simulink model "net2"  (R2014b)
settings: Solver=ode23tb  SolverMode=SingleTasking  StartTime=0.0  StopTime=0.06  RelTol=1e-4
libraries: powerlib x14
Description:
  | Copyright 2008-2014 The MathWorks, Inc.
settings Model: ExtModeTrigMode=oneshot  ExtModeArmWhenConnect=off  ExtModeAutoUpdateStatusClock=off  Creator=MathWorks  LastModifiedBy=jmmauricio
settings SolverCC: ZeroCrossAlgorithm=Adaptive
settings DataIOCC: LimitDataPoints=off  SignalLoggingSaveFormat=ModelDataLogs  SignalLoggingName=sigsOut
settings OptimizationCC: BooleanDataType=off  ExpressionDepthLimit=2147483647  InitFltsAndDblsToZero=on  EfficientMapNaN2IntZero=off
settings DebuggingCC: SaveWithParameterizedLinksMsg=none  UnderspecifiedInitializationDetection=Classic  MergeDetectMultiDrivingBlocksExec=none  SignalResolutionControl=TryResolveAllWithWarning  SolverPrmCheckMsg=none  MultiTaskDSMMsg=warning  MultiTaskCondExecSysMsg=none  SigSpecEnsureSampleTimeMsg=none  FcnCallInpInsideContextMsg=UseLocalSettings  StateNameClashWarn=warning
settings HardwareCC: TargetUnknown=on
settings RTWCC: IncludeERTFirstTime=on
settings GRTTargetCC: TargetFcnLib=ansi_tfl_tmw.mat  CombineOutputUpdateFcns=off  GRTInterface=on

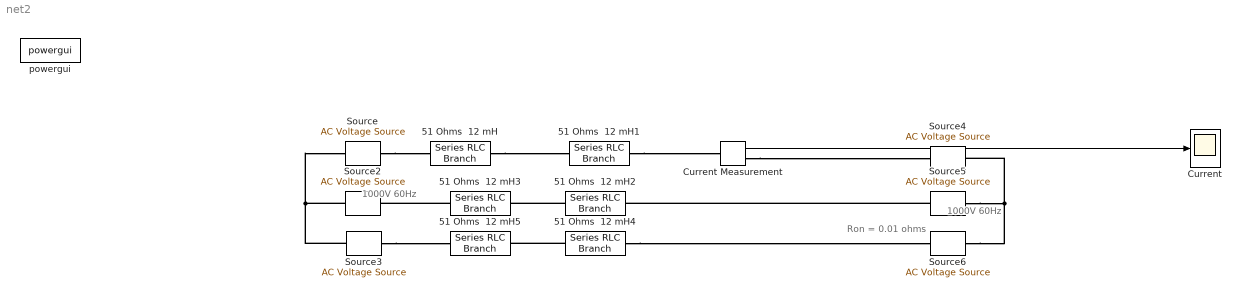
== system net2 ==
  note: Ron = 0.01 ohms
  note: 1000V
      |  60Hz
  note: 1000V
      |  60Hz
  51 Ohms  12 mH{,1..2,5} (4 alike) : powerlib/Elements/Series RLC Branch  LConnTagsString=__new0  RConnTagsString=__new0  BranchType=RL  Resistance=51  Inductance=12e-03  SetiL0=off  InitialCurrent=0  Capacitance=[]  Setx0=off  InitialVoltage=0  Measurements=None
  51 Ohms  12 mH3 : powerlib/Elements/Series RLC Branch  LConnTagsString=__new0  RConnTagsString=__new0  BranchType=RL  Resistance=2  Inductance=12e-03  SetiL0=off  InitialCurrent=0  Capacitance=[]  Setx0=off  InitialVoltage=0  Measurements=None
  51 Ohms  12 mH4 : powerlib/Elements/Series RLC Branch  LConnTagsString=__new0  RConnTagsString=__new0  BranchType=RL  Resistance=51  Inductance=50e-03  SetiL0=off  InitialCurrent=0  Capacitance=[]  Setx0=off  InitialVoltage=0  Measurements=None
  Current : Scope
      settings: TickLabels=on  TimeRange=0.06  YMin=-20  YMax=20
  Current Measurement : powerlib/Measurements/Current Measurement  Tag=PoWeRsYsTeMmEaSuReMeNt  PhasorSimulation=off  OutputType=Magnitude  PSBequivalent=0
  Source{,2..6} (6 alike) : powerlib/Electrical Sources/AC Voltage Source  Description=source block  Amplitude=1000  Phase=0  Frequency=60  SampleTime=0  Measurements=None
      settings: AttributesFormatString=\n
  powergui : powerlib/powergui  SimulationMode=Continuous  SolverType=Tustin  SampleTime=0  frequency=60  SPID=off  DisableSnubberDevices=off  DisableRonSwitches=off  DisableVfSwitches=off  SwTol=0  DisplayEquations=off  Interpol=off  methode=off  Ts=0  frequencyindice=60  Pbase=100e6  ErrMax=1e-4  Iterations=50  UnitsV=kV  UnitsW=MW  FunctionMessages=off  echomessages=off  HookPort=off  EnableUseOfTLC=off  x0status=blocks  RestoreLinks=warning  ResistiveCurrentMeasurement=off  Frange=[0:2:500]  Ylog=off  Xlog=on  ShowGrid=off  save=off  variable=ZData  structure=0  ZoomFFT=on  StartTime=0.0  cycles=1  DisplayStyle=1  fundamental=60  FreqAxis=off  MaxFrequency=1000  frequencyindicesteady=1  RmsSteady=1  display=off
  wires:
  Current Measurement/1 -> Current/1
  connections:
  51 Ohms  12 mH1/RConn1 -- Current Measurement/LConn1
  Current Measurement/RConn1 -- Source4/RConn1
  Source/RConn1 -- 51 Ohms  12 mH/LConn1
  51 Ohms  12 mH3/LConn1 -- Source2/RConn1
  51 Ohms  12 mH/RConn1 -- 51 Ohms  12 mH1/LConn1
  51 Ohms  12 mH2/LConn1 -- 51 Ohms  12 mH3/RConn1
  Source3/LConn1 -- Source2/LConn1 -- Source/LConn1
  51 Ohms  12 mH4/LConn1 -- 51 Ohms  12 mH5/RConn1
  Source3/RConn1 -- 51 Ohms  12 mH5/LConn1
  Source5/LConn1 -- Source6/LConn1 -- Source4/LConn1
  Source5/RConn1 -- 51 Ohms  12 mH2/RConn1
  51 Ohms  12 mH4/RConn1 -- Source6/RConn1
